simulink model "flamepropagation"  (R2022b)
settings: Solver=ode45  StartTime=0.0  StopTime=2e4  FixedStep=100  RelTol=1e-3  EnableMultiTasking=on
StartFcn:
  | cput=cputime;
StopFcn:
  | disp('CPU Time Elapsed:');cputime-cput
Description:
  | File Name:  flamepropagation
  | 
  | Purpose:  Illustration of a stiff system
  | 
  | Details:
  | 
  | A model of flame propagation provides an example. This example was derived
  | by Larry Shampine, one of the authors of the MATLAB ODE suite. When you
  | light a match, the ball of flame grows rapidly until it reaches a critical
  | size. Then it remains at that size because the amount of oxygen being
  | consumed by the combustion in the interior of the ball balances the amount
  | available through the surface. The simple model is
  | 
  | ydot = y^2 * ( 1 - y )
  | 
  | This problem is not stiff initially. It only becomes stiff as the solution
  | approaches steady state. This is because the steady-state solution is so
  | "rigid." Any solution near y(t) = 1 increases or decreases rapidly toward
  | that solution. "Rapidly" here is with respect to an unusually long time
  | scale.
  | 
  | You will see that it takes a longer time and uses more timesteps to solve this
  | problem using a non-stiff solver such as ode45 compared to a stiff solver such
  | as ode23s.
settings Model: Creator=nicholas  LastModifiedBy=bensweet
settings SolverCC: AlgebraicLoopSolver=TrustRegion
settings DataIOCC: SaveFormat=Array  ReturnWorkspaceOutputs=off
settings OptimizationCC: BlockReduction=off  BooleanDataType=off  ExpressionDepthLimit=2147483647  InitFltsAndDblsToZero=on  LifeSpan=inf
settings DebuggingCC: UnconnectedInputMsg=warning  UnconnectedOutputMsg=warning  UnconnectedLineMsg=warning  PregeneratedLibrarySubsystemCodeDiagnostic=none  SFMachineParentedDataDiag=warning
settings HardwareCC: ProdBitPerPointer=32  ProdBitPerSizeT=32  ProdBitPerPtrDiffT=32  ProdLargestAtomicFloat=None  ProdIntDivRoundTo=Undefined  ProdEndianess=Unspecified  ProdWordSize=32  ProdHWDeviceType=32-bit Generic  TargetUnknown=on
settings ModelReferenceCC: EnableRefExpFcnMdlSchedulingChecks=on  PropagateSignalLabelsOutOfModel=off
settings SFSimCC: SimUseLocalCustomCode=off
settings RTWCC: RTWUseLocalCustomCode=off  DLArmComputeVersion=19.05
settings CodeAppCC: StateflowObjectComments=on
settings GRTTargetCC: TargetFcnLib=ansi_tfl_tmw.mat  TargetLangStandard=C89/C90 (ANSI)  CombineOutputUpdateFcns=off  GRTInterface=on
settings ConfigComp: CovMetricSettings=dw  CovSaveCumulativeToWorkspaceVar=on  CovSaveSingleToWorkspaceVar=on  CovExternalEMLEnable=off  CovSFcnEnable=off

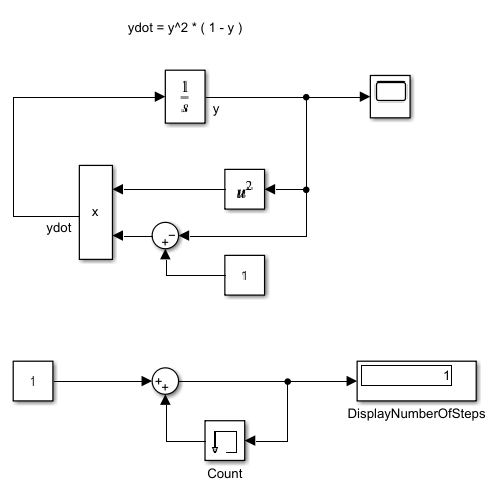
[thumbnail: Simulink's stored preview of the top-level diagram]
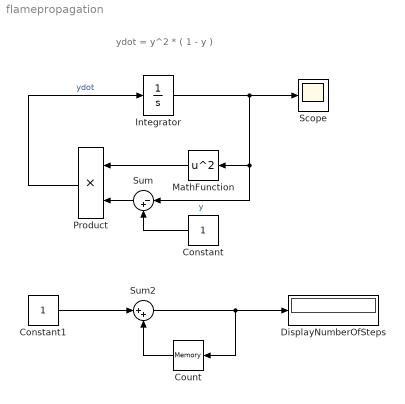
== system flamepropagation ==
  note: ydot = y^2 * ( 1 - y )
  Constant : Constant
  Constant1 : Constant
  Count : Memory
  DisplayNumberOfSteps : Display
  Integrator : Integrator  InitialCondition=1e-4
  MathFunction : Math  Operator=square  SignedPower=on
  Product : Product  InputSameDT=on  RndMeth=Zero  SaturateOnIntegerOverflow=on  OutDataTypeStr=Inherit: Same as first input
  Scope : Scope
  Sum : Sum  Inputs=|-+  InputSameDT=on  SaturateOnIntegerOverflow=on  OutDataTypeStr=Inherit: Same as first input
  Sum2 : Sum  Inputs=|++  InputSameDT=on  SaturateOnIntegerOverflow=on  OutDataTypeStr=Inherit: Same as first input
  wires:
  MathFunction/1 -> Product/1
  Product/1 -> Integrator/1  "ydot"
  Constant/1 -> Sum/2
  Sum/1 -> Product/2
  Integrator/1 -> MathFunction/1, Sum/1, Scope/1  "y"
  Constant1/1 -> Sum2/1
  Sum2/1 -> DisplayNumberOfSteps/1, Count/1
  Count/1 -> Sum2/2
